simulink subsystem "Stewart_Platform_no_sensors"  (R2019b)
settings: Solver=VariableStepAuto  StartTime=0.0  StopTime=10.0  RelTol=1e-3
settings Model: Creator=thomas  LastModifiedBy=thomas

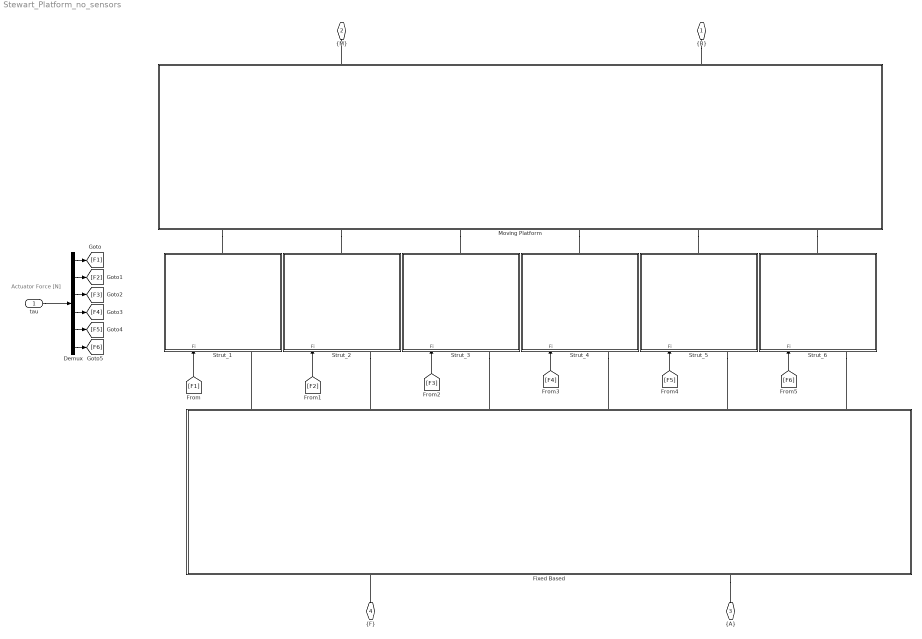
== system Stewart_Platform_no_sensors ==
  note: Actuator Force [N]
  tau : Inport
  Demux : Demux  Outputs=6
  Fixed Based : Subsystem  ReferencedSubsystem=Fixed_Based
  Moving Platform : Subsystem  ReferencedSubsystem=Mobile_Platform
  Strut_1 : Subsystem
      mask init:
      | i=1;
  Strut_2 : Subsystem
      mask init:
      | i=2;
  Strut_3 : Subsystem
      mask init:
      | i=3;
  Strut_4 : Subsystem
      mask init:
      | i=4;
  Strut_5 : Subsystem
      mask init:
      | i=5;
  Strut_6 : Subsystem
      mask init:
      | i=6;
  "{B}" : PMIOPort  Side=Right
  "{M}" : PMIOPort  Port=2  Side=Right
  "{A}" : PMIOPort  Port=3  Side=Left
  "{F}" : PMIOPort  Port=4  Side=Left
  wires:
  [F3] -> Strut_3/1(Fi)
  [F4] -> Strut_4/1(Fi)
  [F1] -> Strut_1/1(Fi)
  Demux/5 -> [F5]
  Demux/1 -> [F1]
  Demux/6 -> [F6]
  Demux/3 -> [F3]
  Demux/2 -> [F2]
  [F2] -> Strut_2/1(Fi)
  [F5] -> Strut_5/1(Fi)
  [F6] -> Strut_6/1(Fi)
  tau/1 -> Demux/1
  Demux/4 -> [F4]
  connections:
  Strut_5/LConn1 -- Fixed Based/RConn5
  Fixed Based/RConn1 -- Strut_1/LConn1
  Strut_4/LConn1 -- Fixed Based/RConn4
  Strut_3/LConn1 -- Fixed Based/RConn3
  Fixed Based/LConn2 -- "{A}"/RConn1
  "{B}"/RConn1 -- Moving Platform/RConn2
  "{F}"/RConn1 -- Fixed Based/LConn1
  Moving Platform/RConn1 -- "{M}"/RConn1
  Strut_6/LConn1 -- Fixed Based/RConn6
  Strut_2/LConn1 -- Fixed Based/RConn2
  Moving Platform/LConn1 -- Strut_1/RConn1
  Moving Platform/LConn2 -- Strut_2/RConn1
  Moving Platform/LConn3 -- Strut_3/RConn1
  Moving Platform/LConn4 -- Strut_4/RConn1
  Moving Platform/LConn5 -- Strut_5/RConn1
  Moving Platform/LConn6 -- Strut_6/RConn1

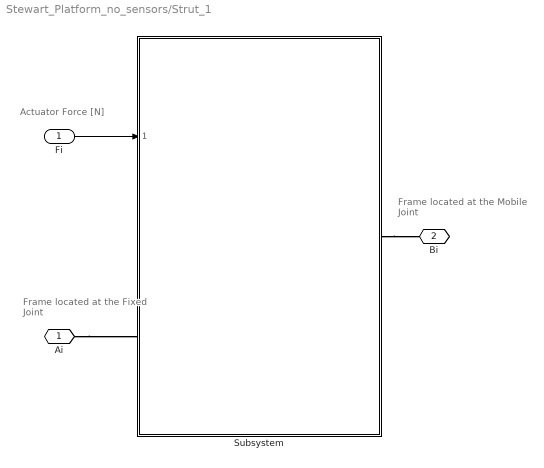
== system Stewart_Platform_no_sensors/Strut_1 ==
  note: Frame located at
      | the Mobile Joint
  note: Actuator Force [N]
  note: Frame located at
      | the Fixed Joint
  Fi : Inport
  Subsystem : Subsystem  VariantControl=with_sensors  ReferencedSubsystem=stewart_strut_no_sensors
  Ai : PMIOPort  Side=Left
  Bi : PMIOPort  Port=2  Side=Right
  wires:
  Fi/1 -> Subsystem/1
  connections:
  Subsystem/RConn1 -- Bi/RConn1
  Ai/RConn1 -- Subsystem/LConn1

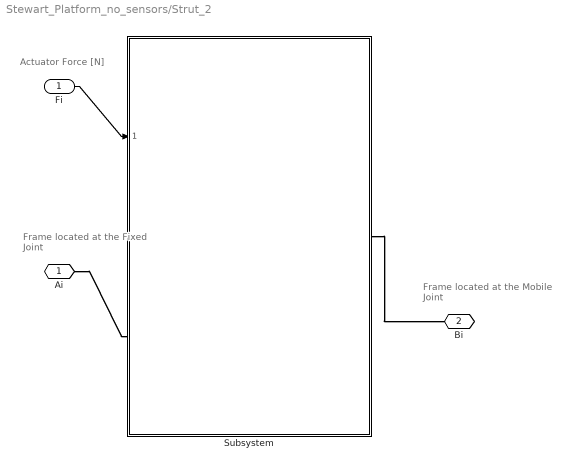
== system Stewart_Platform_no_sensors/Strut_2 ==
  note: Frame located at
      | the Fixed Joint
  note: Actuator Force [N]
  note: Frame located at
      | the Mobile Joint
  Fi : Inport
  Subsystem : Subsystem  VariantControl=with_sensors  ReferencedSubsystem=stewart_strut_no_sensors
  Ai : PMIOPort  Side=Left
  Bi : PMIOPort  Port=2  Side=Right
  wires:
  Fi/1 -> Subsystem/1
  connections:
  Ai/RConn1 -- Subsystem/LConn1
  Subsystem/RConn1 -- Bi/RConn1

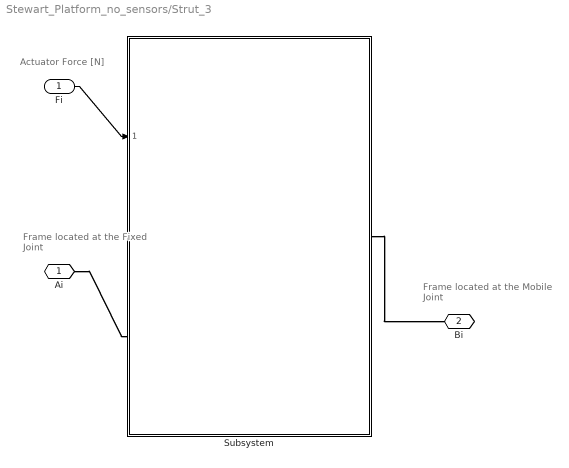
== system Stewart_Platform_no_sensors/Strut_3 ==
  note: Frame located at
      | the Mobile Joint
  note: Actuator Force [N]
  note: Frame located at
      | the Fixed Joint
  Fi : Inport
  Subsystem : Subsystem  VariantControl=with_sensors  ReferencedSubsystem=stewart_strut_no_sensors
  Ai : PMIOPort  Side=Left
  Bi : PMIOPort  Port=2  Side=Right
  wires:
  Fi/1 -> Subsystem/1
  connections:
  Subsystem/RConn1 -- Bi/RConn1
  Ai/RConn1 -- Subsystem/LConn1

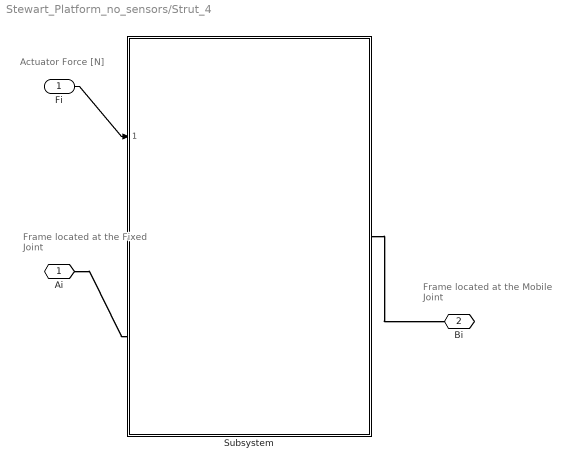
== system Stewart_Platform_no_sensors/Strut_4 ==
  note: Frame located at
      | the Fixed Joint
  note: Actuator Force [N]
  note: Frame located at
      | the Mobile Joint
  Fi : Inport
  Subsystem : Subsystem  VariantControl=with_sensors  ReferencedSubsystem=stewart_strut_no_sensors
  Ai : PMIOPort  Side=Left
  Bi : PMIOPort  Port=2  Side=Right
  wires:
  Fi/1 -> Subsystem/1
  connections:
  Ai/RConn1 -- Subsystem/LConn1
  Subsystem/RConn1 -- Bi/RConn1

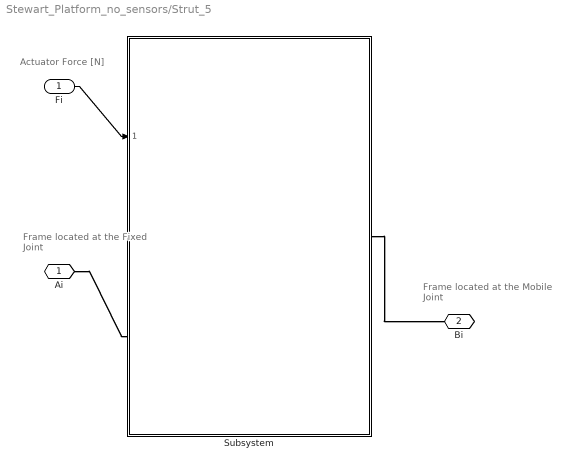
== system Stewart_Platform_no_sensors/Strut_5 ==
  note: Frame located at
      | the Mobile Joint
  note: Actuator Force [N]
  note: Frame located at
      | the Fixed Joint
  Fi : Inport
  Subsystem : Subsystem  VariantControl=with_sensors  ReferencedSubsystem=stewart_strut_no_sensors
  Ai : PMIOPort  Side=Left
  Bi : PMIOPort  Port=2  Side=Right
  wires:
  Fi/1 -> Subsystem/1
  connections:
  Subsystem/RConn1 -- Bi/RConn1
  Ai/RConn1 -- Subsystem/LConn1

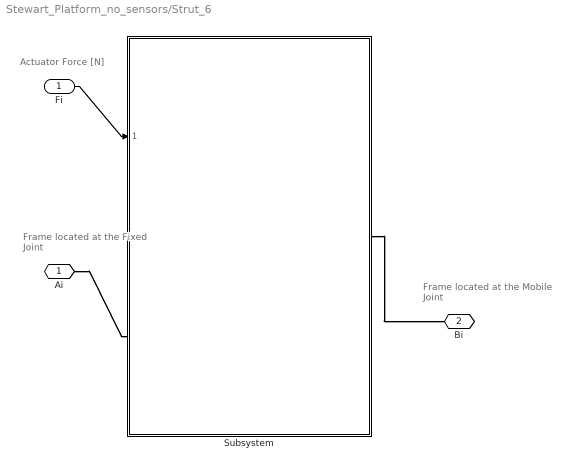
== system Stewart_Platform_no_sensors/Strut_6 ==
  note: Frame located at
      | the Fixed Joint
  note: Actuator Force [N]
  note: Frame located at
      | the Mobile Joint
  Fi : Inport
  Subsystem : Subsystem  VariantControl=with_sensors  ReferencedSubsystem=stewart_strut_no_sensors
  Ai : PMIOPort  Side=Left
  Bi : PMIOPort  Port=2  Side=Right
  wires:
  Fi/1 -> Subsystem/1
  connections:
  Ai/RConn1 -- Subsystem/LConn1
  Subsystem/RConn1 -- Bi/RConn1
